simulink model "Enceinte_climatique_avec_correcteur"  (R2025b)
settings: Solver=VariableStepAuto  StartTime=0.0  StopTime=10.0  RelTol=1e-3
undefined symbols (not defined in the file): dspblkCoreblockFVToolHelper, gcbh
settings Model: Creator=rofte  LastModifiedBy=elio

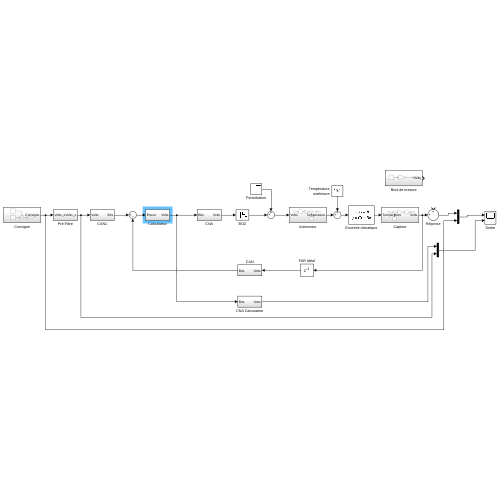
[thumbnail: Simulink's stored preview of the top-level diagram]
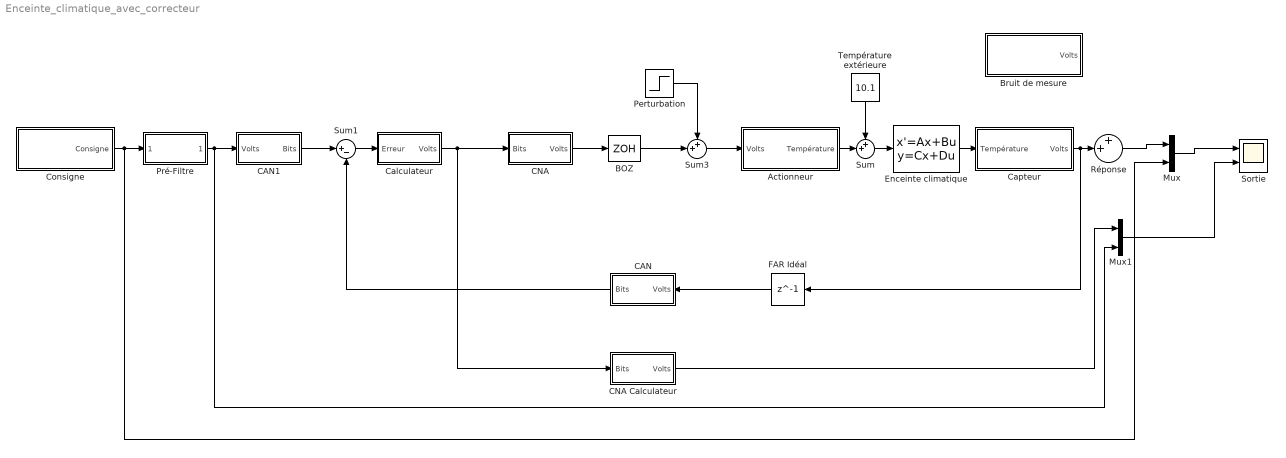
== system Enceinte_climatique_avec_correcteur ==
  Actionneur : Subsystem
  BOZ : ZeroOrderHold  SampleTime=0.01
  Bruit de mesure : Subsystem
  CAN : Subsystem
  CAN1 : Subsystem
  CNA : Subsystem
  CNA Calculateur : Subsystem
  Calculateur : Subsystem
  Capteur : Subsystem
  Consigne : Subsystem
  Enceinte climatique : StateSpace  A=-2  B=2  D=0  InitialCondition=9.95
  FAR Idéal : Delay  DelayLength=1  InitialCondition=0  SampleTime=0.01
  Mux : Mux  Inputs=2
  Mux1 : Mux  Inputs=2
  Perturbation : Step  Time=2  SampleTime=0.01
  Pré-Filtre : Subsystem
  Réponse : Sum  Inputs=++|
  Sortie : Scope  NumInputPorts=2
      settings: ActiveDisplayYMinimum=0.90225149480584443  ActiveDisplayYMaximum=2.8286001569804933
  Sum : Sum  Inputs=++|
  Sum1 : Sum  Inputs=|+-
  Sum3 : Sum  Inputs=++|
  Température extérieure : Constant  Value=10.1
  wires:
  Enceinte climatique/1 -> Capteur/1(Température)
  Capteur/1(Volts) -> FAR Idéal/1, Réponse/2
  Actionneur/1(Température) -> Sum/2
  Sum/1 -> Enceinte climatique/1
  Température extérieure/1 -> Sum/1
  Sum3/1 -> Actionneur/1(Volts)
  Sum1/1 -> Calculateur/1(Erreur)
  Consigne/1(Consigne) -> Pré-Filtre/1(Volts_e), Mux/2
  CAN/1(Bits) -> Sum1/2
  CNA/1(Volts) -> BOZ/1
  Réponse/1 -> Mux/1
  Mux/1 -> Sortie/1
  Mux1/1 -> Sortie/2
  Perturbation/1 -> Sum3/1
  FAR Idéal/1 -> CAN/1(Volts)
  CAN1/1(Bits) -> Sum1/1
  Pré-Filtre/1(Volts_s) -> Mux1/2, CAN1/1(Volts)
  BOZ/1 -> Sum3/2
  CNA Calculateur/1(Volts) -> Mux1/1
  Calculateur/1(Volts) -> CNA/1(Bits), CNA Calculateur/1(Bits)

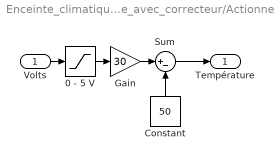
== system Enceinte_climatique_avec_correcteur/Actionneur ==
  Volts : Inport
  "0 - 5 V " : Saturate  UpperLimit=5  LowerLimit=0
  Constant : Constant  Value=50
  Gain : Gain  Gain=30
  Sum : Sum  Inputs=|+-
  Température : Outport
  wires:
  Volts/1 -> "0 - 5 V "/1
  "0 - 5 V "/1 -> Gain/1
  Gain/1 -> Sum/1
  Constant/1 -> Sum/2
  Sum/1 -> Température/1

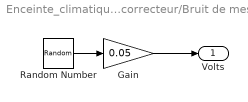
== system Enceinte_climatique_avec_correcteur/Bruit de mesure ==
  Gain : Gain  Gain=0.05
  Random Number : RandomNumber  Variance=0.5  SampleTime=0.01
  Volts : Outport
  wires:
  Random Number/1 -> Gain/1
  Gain/1 -> Volts/1

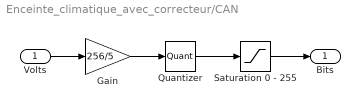
== system Enceinte_climatique_avec_correcteur/CAN ==
  Volts : Inport
  Gain : Gain  Gain=256/5  SaturateOnIntegerOverflow=on  OutDataTypeStr=Inherit: Same as input  ParamDataTypeStr=Inherit: Same as input
  Quantizer : Quantizer  QuantizationInterval=1
  Saturation 0 - 255 : Saturate  UpperLimit=255  LowerLimit=0
  Bits : Outport
  wires:
  Gain/1 -> Quantizer/1
  Volts/1 -> Gain/1
  Quantizer/1 -> Saturation 0 - 255/1
  Saturation 0 - 255/1 -> Bits/1

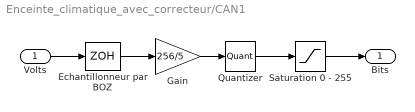
== system Enceinte_climatique_avec_correcteur/CAN1 ==
  Volts : Inport
  Echantillonneur par BOZ : ZeroOrderHold  SampleTime=0.01
  Gain : Gain  Gain=256/5  SaturateOnIntegerOverflow=on  OutDataTypeStr=Inherit: Same as input  ParamDataTypeStr=Inherit: Same as input
  Quantizer : Quantizer  QuantizationInterval=1
  Saturation 0 - 255 : Saturate  UpperLimit=255  LowerLimit=0
  Bits : Outport
  wires:
  Volts/1 -> Echantillonneur par BOZ/1
  Gain/1 -> Quantizer/1
  Echantillonneur par BOZ/1 -> Gain/1
  Quantizer/1 -> Saturation 0 - 255/1
  Saturation 0 - 255/1 -> Bits/1

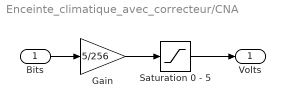
== system Enceinte_climatique_avec_correcteur/CNA ==
  Bits : Inport
  Gain : Gain  Gain=5/256  SaturateOnIntegerOverflow=on  OutDataTypeStr=Inherit: Same as input  ParamDataTypeStr=Inherit: Same as input
  Saturation 0 - 5 : Saturate  UpperLimit=5  LowerLimit=0
  Volts : Outport
  wires:
  Bits/1 -> Gain/1
  Gain/1 -> Saturation 0 - 5/1
  Saturation 0 - 5/1 -> Volts/1

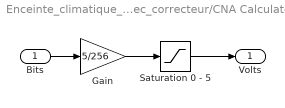
== system Enceinte_climatique_avec_correcteur/CNA Calculateur ==
  Bits : Inport
  Gain : Gain  Gain=5/256  SaturateOnIntegerOverflow=on  OutDataTypeStr=Inherit: Same as input  ParamDataTypeStr=Inherit: Same as input
  Saturation 0 - 5 : Saturate  UpperLimit=5  LowerLimit=0
  Volts : Outport
  wires:
  Bits/1 -> Gain/1
  Gain/1 -> Saturation 0 - 5/1
  Saturation 0 - 5/1 -> Volts/1

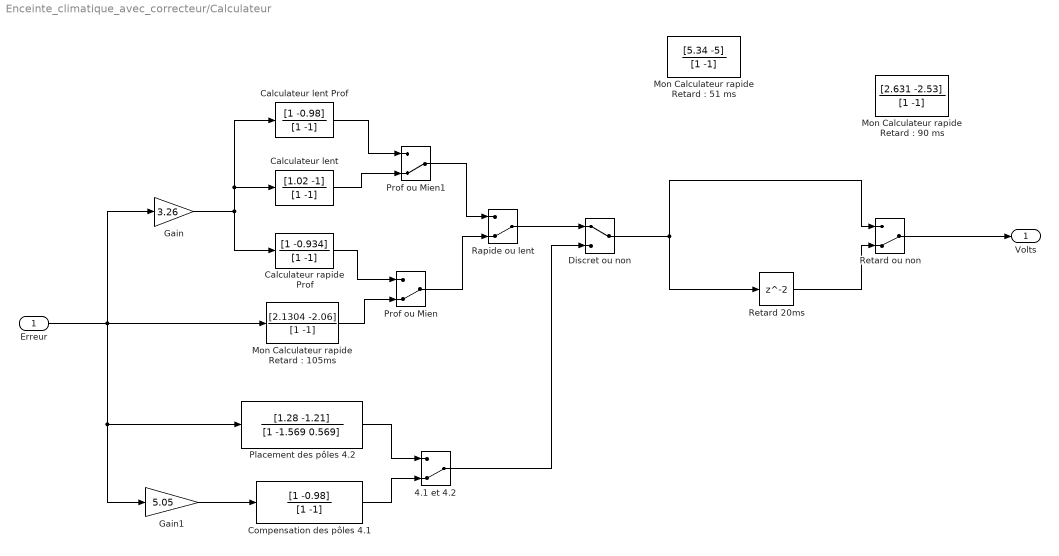
== system Enceinte_climatique_avec_correcteur/Calculateur ==
  Erreur : Inport
  4.1 et 4.2 : ManualSwitch  CurrentSetting=0
  Calculateur lent : DiscreteFilter  LoadFcn=dspblkCoreblockFVToolHelper(gcbh,'load');  Numerator=[1.02 -1]  Denominator=[1 -1]  SampleTime=0.01
      settings: CopyFcn=dspblkCoreblockFVToolHelper(gcbh,'copy');  DeleteFcn=dspblkCoreblockFVToolHelper(gcbh,'close');  ModelCloseFcn=dspblkCoreblockFVToolHelper(gcbh,'close');  PreSaveFcn=dspblkCoreblockFVToolHelper(gcbh,'presave');  PostSaveFcn=dspblkCoreblockFVToolHelper(gcbh,'postsave');  CloseFcn=dspblkCoreblockFVToolHelper(gcbh,'close');
  Calculateur lent Prof : DiscreteFilter  LoadFcn=dspblkCoreblockFVToolHelper(gcbh,'load');  Numerator=[1 -0.98]  Denominator=[1 -1]  SampleTime=0.01
      settings: CopyFcn=dspblkCoreblockFVToolHelper(gcbh,'copy');  DeleteFcn=dspblkCoreblockFVToolHelper(gcbh,'close');  ModelCloseFcn=dspblkCoreblockFVToolHelper(gcbh,'close');  PreSaveFcn=dspblkCoreblockFVToolHelper(gcbh,'presave');  PostSaveFcn=dspblkCoreblockFVToolHelper(gcbh,'postsave');  CloseFcn=dspblkCoreblockFVToolHelper(gcbh,'close');
  Calculateur rapide Prof : DiscreteFilter  LoadFcn=dspblkCoreblockFVToolHelper(gcbh,'load');  Numerator=[1 -0.934]  Denominator=[1 -1]  SampleTime=0.01
      settings: CopyFcn=dspblkCoreblockFVToolHelper(gcbh,'copy');  DeleteFcn=dspblkCoreblockFVToolHelper(gcbh,'close');  ModelCloseFcn=dspblkCoreblockFVToolHelper(gcbh,'close');  PreSaveFcn=dspblkCoreblockFVToolHelper(gcbh,'presave');  PostSaveFcn=dspblkCoreblockFVToolHelper(gcbh,'postsave');  CloseFcn=dspblkCoreblockFVToolHelper(gcbh,'close');
  Compensation des pôles 4.1 : DiscreteFilter  LoadFcn=dspblkCoreblockFVToolHelper(gcbh,'load');  Numerator=[1 -0.98]  Denominator=[1 -1]  SampleTime=0.01
      settings: CopyFcn=dspblkCoreblockFVToolHelper(gcbh,'copy');  DeleteFcn=dspblkCoreblockFVToolHelper(gcbh,'close');  ModelCloseFcn=dspblkCoreblockFVToolHelper(gcbh,'close');  PreSaveFcn=dspblkCoreblockFVToolHelper(gcbh,'presave');  PostSaveFcn=dspblkCoreblockFVToolHelper(gcbh,'postsave');  CloseFcn=dspblkCoreblockFVToolHelper(gcbh,'close');
  Discret ou non : ManualSwitch
  Gain : Gain  Gain=3.26
  Gain1 : Gain  Gain=5.05
  "Mon Calculateur rapide Retard : 105ms" : DiscreteFilter  LoadFcn=dspblkCoreblockFVToolHelper(gcbh,'load');  Numerator=[2.1304 -2.06]  Denominator=[1 -1]  SampleTime=0.01
      settings: CopyFcn=dspblkCoreblockFVToolHelper(gcbh,'copy');  DeleteFcn=dspblkCoreblockFVToolHelper(gcbh,'close');  ModelCloseFcn=dspblkCoreblockFVToolHelper(gcbh,'close');  PreSaveFcn=dspblkCoreblockFVToolHelper(gcbh,'presave');  PostSaveFcn=dspblkCoreblockFVToolHelper(gcbh,'postsave');  CloseFcn=dspblkCoreblockFVToolHelper(gcbh,'close');
  "Mon Calculateur rapide Retard : 51 ms" : DiscreteFilter  LoadFcn=dspblkCoreblockFVToolHelper(gcbh,'load');  Numerator=[5.34 -5]  Denominator=[1 -1]  SampleTime=0.01
      settings: CopyFcn=dspblkCoreblockFVToolHelper(gcbh,'copy');  DeleteFcn=dspblkCoreblockFVToolHelper(gcbh,'close');  ModelCloseFcn=dspblkCoreblockFVToolHelper(gcbh,'close');  PreSaveFcn=dspblkCoreblockFVToolHelper(gcbh,'presave');  PostSaveFcn=dspblkCoreblockFVToolHelper(gcbh,'postsave');  CloseFcn=dspblkCoreblockFVToolHelper(gcbh,'close');
  "Mon Calculateur rapide Retard : 90 ms" : DiscreteFilter  LoadFcn=dspblkCoreblockFVToolHelper(gcbh,'load');  Numerator=[2.631 -2.53]  Denominator=[1 -1]  SampleTime=0.01
      settings: CopyFcn=dspblkCoreblockFVToolHelper(gcbh,'copy');  DeleteFcn=dspblkCoreblockFVToolHelper(gcbh,'close');  ModelCloseFcn=dspblkCoreblockFVToolHelper(gcbh,'close');  PreSaveFcn=dspblkCoreblockFVToolHelper(gcbh,'presave');  PostSaveFcn=dspblkCoreblockFVToolHelper(gcbh,'postsave');  CloseFcn=dspblkCoreblockFVToolHelper(gcbh,'close');
  Placement des pôles 4.2 : DiscreteFilter  LoadFcn=dspblkCoreblockFVToolHelper(gcbh,'load');  Numerator=[1.28 -1.21]  Denominator=[1 -1.569 0.569]  SampleTime=0.01
      settings: CopyFcn=dspblkCoreblockFVToolHelper(gcbh,'copy');  DeleteFcn=dspblkCoreblockFVToolHelper(gcbh,'close');  ModelCloseFcn=dspblkCoreblockFVToolHelper(gcbh,'close');  PreSaveFcn=dspblkCoreblockFVToolHelper(gcbh,'presave');  PostSaveFcn=dspblkCoreblockFVToolHelper(gcbh,'postsave');  CloseFcn=dspblkCoreblockFVToolHelper(gcbh,'close');
  Prof ou Mien : ManualSwitch  CurrentSetting=0
  Prof ou Mien1 : ManualSwitch  CurrentSetting=0
  Rapide ou lent : ManualSwitch  CurrentSetting=0
  Retard 20ms : Delay  InitialCondition=0  SampleTime=0.01
  Retard ou non : ManualSwitch  CurrentSetting=0
  Volts : Outport
  wires:
  Erreur/1 -> "Mon Calculateur rapide Retard : 105ms"/1, Gain/1, Gain1/1, Placement des pôles 4.2/1
  Gain/1 -> Calculateur rapide Prof/1, Calculateur lent/1, Calculateur lent Prof/1
  "Mon Calculateur rapide Retard : 105ms"/1 -> Prof ou Mien/2
  Calculateur rapide Prof/1 -> Prof ou Mien/1
  Prof ou Mien/1 -> Rapide ou lent/2
  Rapide ou lent/1 -> Discret ou non/1
  Gain1/1 -> Compensation des pôles 4.1/1
  Compensation des pôles 4.1/1 -> 4.1 et 4.2/2
  Placement des pôles 4.2/1 -> 4.1 et 4.2/1
  4.1 et 4.2/1 -> Discret ou non/2
  Discret ou non/1 -> Retard ou non/1, Retard 20ms/1
  Retard ou non/1 -> Volts/1
  Retard 20ms/1 -> Retard ou non/2
  Prof ou Mien1/1 -> Rapide ou lent/1
  Calculateur lent Prof/1 -> Prof ou Mien1/1
  Calculateur lent/1 -> Prof ou Mien1/2

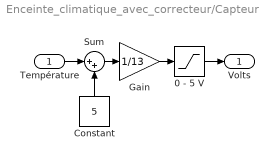
== system Enceinte_climatique_avec_correcteur/Capteur ==
  Température : Inport
  "0 - 5 V " : Saturate  UpperLimit=5  LowerLimit=0
  Constant : Constant  Value=5
  Gain : Gain  Gain=1/13
  Sum : Sum  Inputs=|++
  Volts : Outport
  wires:
  Constant/1 -> Sum/2
  Température/1 -> Sum/1
  Sum/1 -> Gain/1
  Gain/1 -> "0 - 5 V "/1
  "0 - 5 V "/1 -> Volts/1

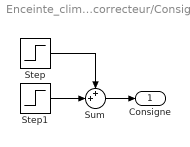
== system Enceinte_climatique_avec_correcteur/Consigne ==
  Step : Step  Time=4  After=-0.5  SampleTime=0.01
  Step1 : Step  Time=0.5  Before=1.66  After=2.33  SampleTime=0.01
  Sum : Sum  Inputs=++|
  Consigne : Outport
  wires:
  Step/1 -> Sum/1
  Step1/1 -> Sum/2
  Sum/1 -> Consigne/1

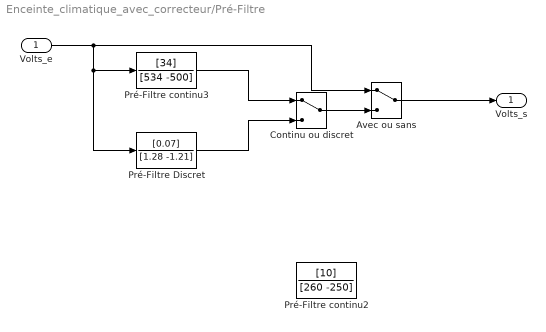
== system Enceinte_climatique_avec_correcteur/Pré-Filtre ==
  Volts_e : Inport
  Avec ou sans : ManualSwitch
  Continu ou discret : ManualSwitch
  Pré-Filtre Discret : DiscreteFilter  LoadFcn=dspblkCoreblockFVToolHelper(gcbh,'load');  Numerator=[0.07]  Denominator=[1.28 -1.21]  SampleTime=0.01
      settings: CopyFcn=dspblkCoreblockFVToolHelper(gcbh,'copy');  DeleteFcn=dspblkCoreblockFVToolHelper(gcbh,'close');  ModelCloseFcn=dspblkCoreblockFVToolHelper(gcbh,'close');  PreSaveFcn=dspblkCoreblockFVToolHelper(gcbh,'presave');  PostSaveFcn=dspblkCoreblockFVToolHelper(gcbh,'postsave');  CloseFcn=dspblkCoreblockFVToolHelper(gcbh,'close');
  Pré-Filtre continu2 : DiscreteFilter  LoadFcn=dspblkCoreblockFVToolHelper(gcbh,'load');  Numerator=[10]  Denominator=[260 -250]  SampleTime=0.01
      settings: CopyFcn=dspblkCoreblockFVToolHelper(gcbh,'copy');  DeleteFcn=dspblkCoreblockFVToolHelper(gcbh,'close');  ModelCloseFcn=dspblkCoreblockFVToolHelper(gcbh,'close');  PreSaveFcn=dspblkCoreblockFVToolHelper(gcbh,'presave');  PostSaveFcn=dspblkCoreblockFVToolHelper(gcbh,'postsave');  CloseFcn=dspblkCoreblockFVToolHelper(gcbh,'close');
  Pré-Filtre continu3 : DiscreteFilter  LoadFcn=dspblkCoreblockFVToolHelper(gcbh,'load');  Numerator=[34]  Denominator=[534 -500]  SampleTime=0.01
      settings: CopyFcn=dspblkCoreblockFVToolHelper(gcbh,'copy');  DeleteFcn=dspblkCoreblockFVToolHelper(gcbh,'close');  ModelCloseFcn=dspblkCoreblockFVToolHelper(gcbh,'close');  PreSaveFcn=dspblkCoreblockFVToolHelper(gcbh,'presave');  PostSaveFcn=dspblkCoreblockFVToolHelper(gcbh,'postsave');  CloseFcn=dspblkCoreblockFVToolHelper(gcbh,'close');
  Volts_s : Outport
  wires:
  Volts_e/1 -> Pré-Filtre continu3/1, Pré-Filtre Discret/1, Avec ou sans/1
  Avec ou sans/1 -> Volts_s/1
  Pré-Filtre continu3/1 -> Continu ou discret/1
  Continu ou discret/1 -> Avec ou sans/2
  Pré-Filtre Discret/1 -> Continu ou discret/2
